simulink subsystem "INA219_Current_Sensor"  (R2022b)
settings: Solver=VariableStepAuto  StartTime=0.0  StopTime=10.0  RelTol=1e-3
settings Model: Creator=gotta  LastModifiedBy=gotta

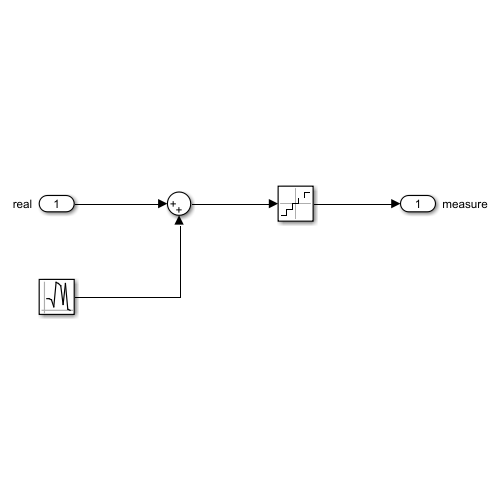
[thumbnail: Simulink's stored preview of the top-level diagram]
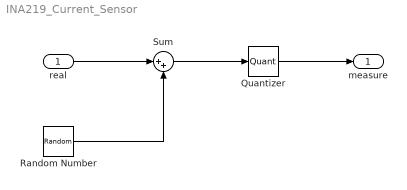
== system INA219_Current_Sensor ==
  real : Inport
  Quantizer : Quantizer  QuantizationInterval=INA219.Istep
  Random Number : RandomNumber  Variance=3e-2  SampleTime=1e-3
  Sum : Sum  Inputs=|++
  measure : Outport
  wires:
  Sum/1 -> Quantizer/1
  Quantizer/1 -> measure/1
  Random Number/1 -> Sum/2
  real/1 -> Sum/1
